simulink model "APV_T"  (R2021a)
settings: Solver=VariableStepAuto  StartTime=0.0  StopTime=Duration  RelTol=1e-3
values from neighbouring files (symbols this model uses):
  Ts = 0.1    [createMPCForTrackingParkingValet.m]
undefined symbols (not defined in the file or in its folder): info, pTracking
libraries: robotmobilelib x1, mpclib x1, simulink_extras x1
settings Model: Creator=The MathWorks, Inc.  LastModifiedBy=jiaya
settings SolverCC: AlgebraicLoopSolver=TrustRegion
settings DebuggingCC: SFMachineParentedDataDiag=warning

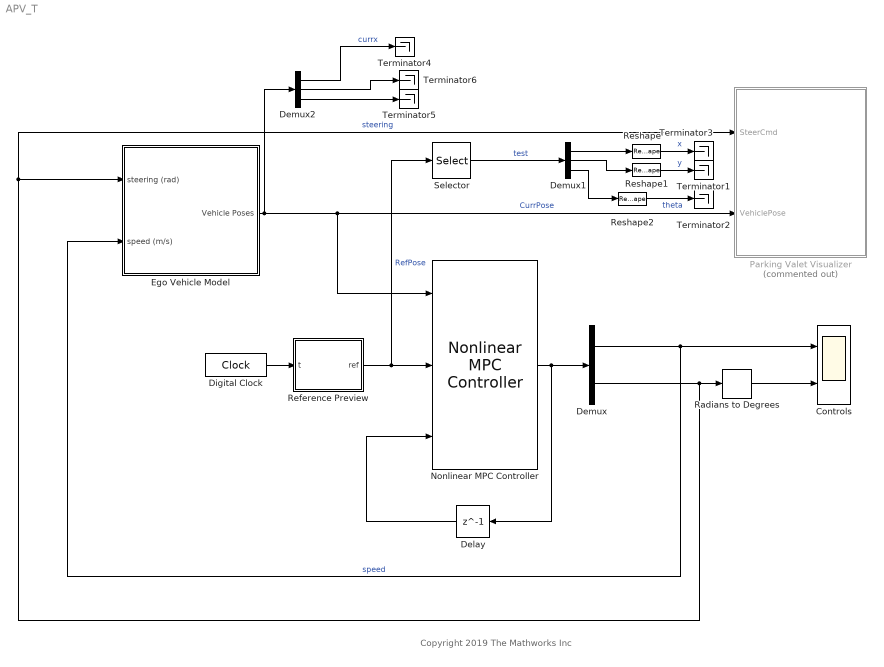
== system APV_T ==
  note: Copyright 2019 The Mathworks Inc
  Controls : Scope  NumInputPorts=2
  Delay : Delay  DelayLength=1
  Demux : Demux  Outputs=[1 1]
  Demux1 : Demux  Outputs=3
  Demux2 : Demux  Outputs=3
  Digital Clock : DigitalClock  SampleTime=Ts
  Ego Vehicle Model : Subsystem
  Nonlinear MPC Controller : mpclib/Nonlinear MPC Controller  SCDEnableBlockLinearizationSpecification=on  nlmpcobj=nlobjTracking  UseObjectTs=on  UseMEX=off  mexname=''  md_enabled=off  mvtarget_enabled=off  param_enabled=off  cost_enabled=off  mvseq_enabled=off  stateseq_enabled=off  ovseq_enabled=off  slack_enabled=off  status_enabled=off  ov_min=off  ov_max=off  mv_min=off  mv_max=off  mvrate_min=off  mvrate_max=off  state_min=off  state_max=off  ov_weight=off  mv_weight=off  mvrate_weight=off  ecr_weight=off  nlp_initialize=off
  Parking Valet Visualizer : Subsystem  Commented=on
  Radians to Degrees : simulink_extras/Transformations/Radians to Degrees
  Reference Preview : MATLAB Function  TreatAsAtomicUnit=on
  Reshape : Reshape  OutputDimensionality=Customize  OutputDimensions=[1]
  Reshape1 : Reshape  OutputDimensionality=Customize  OutputDimensions=[1]
  Reshape2 : Reshape  OutputDimensionality=Customize  OutputDimensions=[1]
  Selector : Selector  NumberOfDimensions=2  InputPortWidth=3  IndexOptions=Index vector (dialog),Index vector (dialog)  Indices=1,[1:3]  OutputSizes=1,1
  Terminator{1..6} (6 alike) : Terminator
  wires:
  Delay/1 -> Nonlinear MPC Controller/3
  Nonlinear MPC Controller/1 -> Delay/1, Demux/1
  Reference Preview/1(ref) -> Selector/1, Nonlinear MPC Controller/2  "RefPose"
  Radians to Degrees/1 -> Controls/2
  Demux/2 -> Radians to Degrees/1, Parking Valet Visualizer/1(SteerCmd), Ego Vehicle Model/1(steering (rad))  "steering"
  Demux/1 -> Ego Vehicle Model/2(speed (m/s)), Controls/1  "speed"
  Digital Clock/1 -> Reference Preview/1(t)
  Ego Vehicle Model/1(Vehicle Poses) -> Parking Valet Visualizer/2(VehiclePose), Nonlinear MPC Controller/1, Demux2/1  "CurrPose"
  Selector/1 -> Demux1/1  "test"
  Demux1/1 -> Reshape/1
  Demux1/2 -> Reshape1/1
  Reshape/1 -> Terminator3/1  "x"
  Reshape1/1 -> Terminator1/1  "y"
  Demux1/3 -> Reshape2/1
  Reshape2/1 -> Terminator2/1  "theta"
  Demux2/1 -> Terminator4/1  "currx"
  Demux2/3 -> Terminator5/1
  Demux2/2 -> Terminator6/1

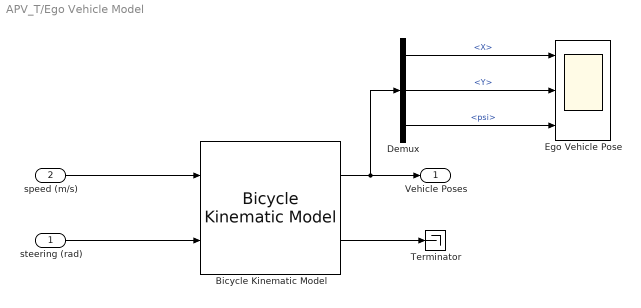
== system APV_T/Ego Vehicle Model ==
  steering (rad) : Inport
  speed (m/s) : Inport  Port=2
  Bicycle Kinematic Model : robotmobilelib/Bicycle Kinematic Model  VehicleInputs=Vehicle Speed & Steering Angle  WheelBase=2.8  VehicleSpeedRange=[-6.5 6.5]  MaxSteeringAngle=pi/4  InitialState=egoInitialPose  SimulateUsing=Interpreted execution
      settings: SourceProductBaseCode=RO
  Demux : Demux  Outputs=3
  Ego Vehicle Pose : Scope  NumInputPorts=3
  Terminator : Terminator
  Vehicle Poses : Outport
  wires:
  Bicycle Kinematic Model/1 -> Demux/1, Vehicle Poses/1
  speed (m/s)/1 -> Bicycle Kinematic Model/1
  steering (rad)/1 -> Bicycle Kinematic Model/2
  Bicycle Kinematic Model/2 -> Terminator/1
  Demux/3 -> Ego Vehicle Pose/3  "<psi>"
  Demux/2 -> Ego Vehicle Pose/2  "<Y>"
  Demux/1 -> Ego Vehicle Pose/1  "<X>"

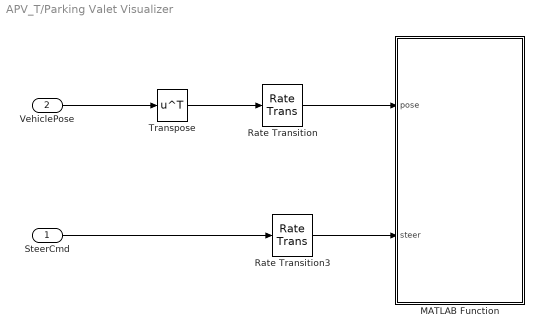
== system APV_T/Parking Valet Visualizer ==
  SteerCmd : Inport
  VehiclePose : Inport  Port=2
  MATLAB Function : MATLAB Function  TreatAsAtomicUnit=on
  Rate Transition : RateTransition  OutPortSampleTime=Tv
  Rate Transition3 : RateTransition  OutPortSampleTime=Tv
  Transpose : Math  Operator=transpose  SaturateOnIntegerOverflow=on
  wires:
  Rate Transition/1 -> MATLAB Function/1(pose)
  VehiclePose/1 -> Transpose/1
  Rate Transition3/1 -> MATLAB Function/2(steer)
  SteerCmd/1 -> Rate Transition3/1
  Transpose/1 -> Rate Transition/1

== matlab function APV_T/Reference Preview ==
  data: t input; ref output; Ts parameter; info parameter; pTracking parameter
function ref = fcn(t,Ts,info,pTracking)
Tend = info.Topt(end);
T = t+(1:pTracking)*Ts;
T = min(T,Tend);
ref = interp1(info.Topt,info.Xopt(:,1:3),T);

== matlab function APV_T/Parking Valet Visualizer/MATLAB Function ==
  data: pose input; steer input; costmapStruct parameter
function visualizeParkingValet(pose, steer, costmapStruct)

%visualizePath Display simulation results.

coder.extrinsic('helperSLVisualizeParkingValet');

helperSLVisualizeParkingValet(pose, steer, costmapStruct);
